simulink model "liner_control"  (R2019b)
settings: Solver=FixedStepAuto  StartTime=0.0  StopTime=100  FixedStep=0.01  RelTol=1e-3
undefined symbols (not defined in the file or in its folder): DiscIntNeverNeededParam
libraries: sbox2 x4, simulink x2
settings Model: Creator=haketa  LastModifiedBy=admin
settings DataIOCC: SaveFormat=Array  SignalLoggingSaveFormat=ModelDataLogs  ReturnWorkspaceOutputs=off
settings OptimizationCC: BlockReduction=off  OptimizeBlockIOStorage=off  BufferReuse=off  GlobalBufferReuse=off  ExpressionFolding=off  ExpressionDepthLimit=2147483647  LocalBlockOutputs=off  InitFltsAndDblsToZero=on  LifeSpan=inf  OptimizeDataStoreBuffers=off  BusAssignmentInplaceUpdate=off
settings DebuggingCC: SaveWithParameterizedLinksMsg=none  UnderspecifiedInitializationDetection=Classic  MergeDetectMultiDrivingBlocksExec=none  SignalResolutionControl=TryResolveAllWithWarning  SolverPrmCheckMsg=warning  InheritedTsInSrcMsg=none  MultiTaskDSMMsg=warning  MultiTaskCondExecSysMsg=none  FcnCallInpInsideContextMsg=warning  StateNameClashWarn=warning  SFUnexpectedBacktrackingDiag=warning  SFNoUnconditionalDefaultTransitionDiag=warning  SFExecutionAtInitializationDiag=none  ArithmeticOperatorsInVariantConditions=warning
settings HardwareCC: ProdBitPerPointer=32  ProdBitPerSizeT=32  ProdBitPerPtrDiffT=32  ProdLargestAtomicFloat=None  ProdIntDivRoundTo=Undefined  ProdEndianess=Unspecified  ProdWordSize=32  ProdHWDeviceType=32-bit Generic
settings ModelReferenceCC: PropagateSignalLabelsOutOfModel=off
settings SFSimCC: SimUseLocalCustomCode=off  CustomCodeUndefinedFunction=UseInterfaceOnly
settings RTWCC: Description=MTT sBOXII Real-Time Target.  SystemTargetFile=sbox2.tlc  TemplateMakefile=sbox2.tmf  RTWUseLocalCustomCode=off  RTWCompilerOptimization=on
settings CodeAppCC: StateflowObjectComments=on
settings GRTTargetCC: TargetLangStandard=C89/C90 (ANSI)  GeneratePreprocessorConditionals=Disable all  MatFileLogging=off  UseToolchainInfoCompliant=off  RTWCAPISignals=on  RTWCAPIParams=on
settings ConfigComp: CovMetricSettings=dw  CovHtmlReporting=on  CovSaveCumulativeToWorkspaceVar=on  CovSaveSingleToWorkspaceVar=on  CovExternalEMLEnable=off  CovSFcnEnable=off

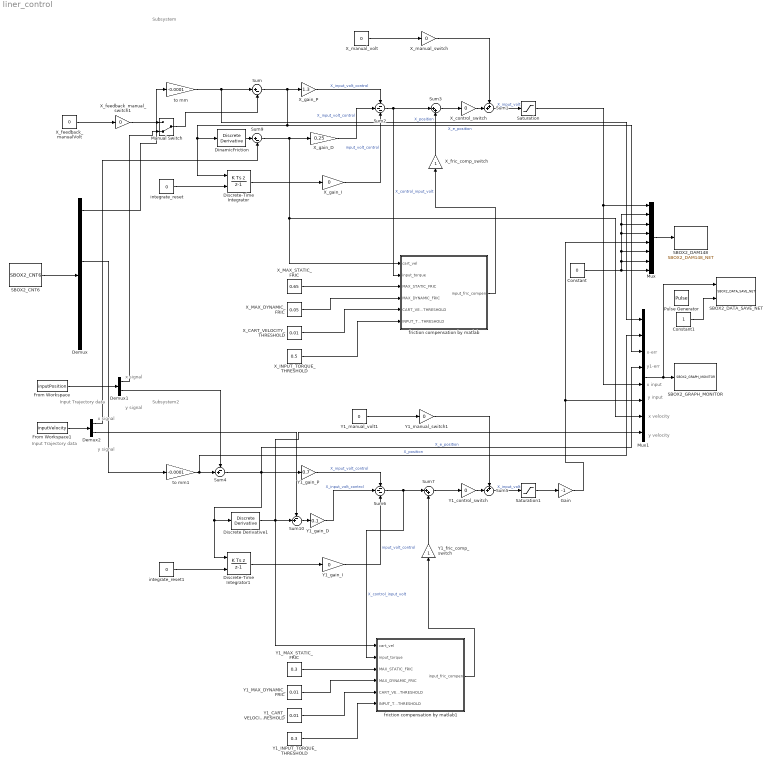
== system liner_control ==
  note: y velocity
  note: x velocity
  note: y input
  note: x input
  note: Input Trajectory data
  note: x signal
  note: y1-err
  note: x-err
  note: Subsystem2
  note: Subsystem
  note: y signal
  note: Input Trajectory data
  note: x signal
  note: y signal
  Constant : Constant  Value=0
  Constant1 : Constant
  Demux : Demux  Outputs=6
  Demux1 : Demux  Outputs=2
  Demux2 : Demux  Outputs=2
  DinamicFriction : simulink/Discrete/Discrete Derivative  gainval=1.0  ICPrevScaledInput=0.0  OutMin=[]  OutMax=[]  OutDataType=fixdt(1, 16)  OutScaling=2^-10  DoSatur=off
  Discrete Derivative1 : simulink/Discrete/Discrete Derivative  gainval=1.0  ICPrevScaledInput=0.0  OutMin=[]  OutMax=[]  OutDataType=fixdt(1, 16)  OutScaling=2^-10  DoSatur=off
  Discrete-Time Integrator : DiscreteIntegrator  IntegratorMethod=Integration: Backward Euler  ExternalReset=rising  SampleTime=-1  ICPrevOutput=DiscIntNeverNeededParam  ICPrevScaledInput=DiscIntNeverNeededParam
  Discrete-Time Integrator1 : DiscreteIntegrator  IntegratorMethod=Integration: Backward Euler  ExternalReset=rising  SampleTime=-1  ICPrevOutput=DiscIntNeverNeededParam  ICPrevScaledInput=DiscIntNeverNeededParam
  From Workspace : FromWorkspace  VariableName=inputPosition  SampleTime=0.01
  From Workspace1 : FromWorkspace  VariableName=inputVelocity  SampleTime=0.01
  Gain : Gain  Gain=-1
  Manual Switch : ManualSwitch  CurrentSetting=0
  Mux : Mux  Inputs=8
  Mux1 : Mux  Inputs=8
  Pulse Generator : DiscretePulseGenerator  Period=100  PulseWidth=5
  SBOX2_CNT6 : sbox2/Digital I//O Devices/SBOX2_CNT6  mode=2相パルス  teibai=x4  filter=off  zphase=動作なし  polarity=正論理 (high active)  mode2=2相パルス  teibai2=x4  filter2=off  zphase2=動作なし  polarity2=正論理 (high active)  mode3=2相パルス  teibai3=x4  filter3=off  zphase3=動作なし  polarity3=正論理 (high active)  mode4=2相パルス  teibai4=x4  filter4=off  zphase4=動作なし  polarity4=正論理 (high active)  mode5=2相パルス  teibai5=x4  filter5=off  zphase5=動作なし  polarity5=正論理 (high active)  mode6=2相パルス  teibai6=x4  filter6=off  zphase6=動作なし  polarity6=正論理 (high active)  dtype=FLOATING POINT  sampletime=-1
  "SBOX2_DAM148 " : sbox2/Analog I//O Devices/SBOX2_DAM148_NET  daStopCtrl1=DA出力継続  daStopCtrl2=DA出力継続  daStopCtrl3=DA出力継続  daStopCtrl4=DA出力継続  daStopCtrl5=DA出力継続  daStopCtrl6=DA出力継続  daStopCtrl7=DA出力継続  daStopCtrl8=DA出力継続  sampletime=-1
  SBOX2_DATA_SAVE_NET : sbox2/Network Data Save Devices/SBOX2_DATA_SAVE_NET  save_mode=ホストアプリケーション指示によるトリガ待ち  data_length=500  pre_triger=0  sampletime=-1
  SBOX2_GRAPH_MONITOR : sbox2/Network Data Save Devices/SBOX2_GRAPH_MONITOR  sampletime=-1
  Saturation : Saturate  UpperLimit=5  LowerLimit=-5
  Saturation1 : Saturate  UpperLimit=5  LowerLimit=-5
  Sum : Sum  Inputs=|+-
  Sum1 : Sum  Inputs=++|
  Sum10 : Sum  Inputs=-+|
  Sum2 : Sum  Inputs=---
  Sum3 : Sum  Inputs=|++
  Sum4 : Sum  Inputs=-+|
  Sum5 : Sum  Inputs=++|
  Sum6 : Sum  Inputs=---
  Sum7 : Sum  Inputs=|++
  Sum9 : Sum  Inputs=|+-
  X_CART_VELOCITY_THRESHOLD : Constant  Value=0.01
  X_INPUT_TORQUE_THRESHOLD : Constant  Value=0.5
  X_MAX_DYNAMIC_FRIC : Constant  Value=0.05
  X_MAX_STATIC_FRIC : Constant  Value=0.65
  X_control_switch : Gain  Gain=0
  X_feedback_manualVolt : Constant  Value=0
  X_feedback_manual_switch1 : Gain  Gain=0
  X_fric_comp_switch : Gain
  X_gain_D : Gain  Gain=0.25
  X_gain_I : Gain  Gain=0
  X_gain_P : Gain  Gain=1.3
  X_manual_switch : Gain  Gain=0
  X_manual_volt : Constant  Value=0
  Y1_CART_VELOCITY_THRESHOLD : Constant  Value=0.01
  Y1_INPUT_TORQUE_THRESHOLD : Constant  Value=0.3
  Y1_MAX_DYNAMIC_FRIC : Constant  Value=0.01
  Y1_MAX_STATIC_FRIC : Constant  Value=0.3
  Y1_control_switch : Gain  Gain=0
  Y1_fric_comp_switch : Gain
  Y1_gain_D : Gain  Gain=0.1
  Y1_gain_I : Gain  Gain=0
  Y1_gain_P : Gain  Gain=0.7
  Y1_manual_switch1 : Gain  Gain=0
  Y1_manual_volt1 : Constant  Value=0
  friction compensation by matlab : MATLAB Function  TreatAsAtomicUnit=on
  friction compensation by matlab1 : MATLAB Function  TreatAsAtomicUnit=on
  integrate_reset : Constant  Value=0
  integrate_reset1 : Constant  Value=0
  to mm : Gain  Gain=-0.0001
  to mm1 : Gain  Gain=-0.0001
  wires:
  SBOX2_CNT6/1 -> Demux/1
  Mux/1 -> "SBOX2_DAM148 "/1
  Constant/1 -> Mux/7, Mux/3, Mux/2, Mux/4, Mux/6, Mux/8
  Saturation/1 -> Mux1/5, Mux/1
  Saturation1/1 -> Gain/1
  X_fric_comp_switch/1 -> Sum3/2
  Sum3/1 -> X_control_switch/1
  X_manual_volt/1 -> X_manual_switch/1
  integrate_reset/1 -> Discrete-Time Integrator/2
  X_CART_VELOCITY_THRESHOLD/1 -> friction compensation by matlab/5(CART_VELOCITY_THRESHOLD)
  X_MAX_DYNAMIC_FRIC/1 -> friction compensation by matlab/4(MAX_DYNAMIC_FRIC)
  to mm/1 -> Mux1/1, Sum/1  "X_position"
  X_gain_D/1 -> Sum2/2  "X_input_volt_control"
  X_MAX_STATIC_FRIC/1 -> friction compensation by matlab/3(MAX_STATIC_FRIC)
  friction compensation by matlab/1(input_fric_compen) -> X_fric_comp_switch/1
  X_manual_switch/1 -> Sum1/1
  X_INPUT_TORQUE_THRESHOLD/1 -> friction compensation by matlab/6(INPUT_TORQUE_THRESHOLD)
  X_gain_I/1 -> Sum2/3  "input_volt_control"
  Sum/1 -> Mux1/3, DinamicFriction/1, Discrete-Time Integrator/1, X_gain_P/1  "X_e_position"
  X_gain_P/1 -> Sum2/1  "X_input_volt_control"
  Discrete-Time Integrator/1 -> X_gain_I/1
  Sum2/1 -> Sum3/1, friction compensation by matlab/2(input_torque)  "X_control_input_volt"
  Demux/1 -> to mm/1
  Sum9/1 -> friction compensation by matlab/1(cart_vel), Mux1/7, X_gain_D/1
  Sum1/1 -> Saturation/1  "X_input_volt"
  Y1_fric_comp_switch/1 -> Sum7/2
  Sum7/1 -> Y1_control_switch/1
  Y1_manual_volt1/1 -> Y1_manual_switch1/1
  integrate_reset1/1 -> Discrete-Time Integrator1/2
  Y1_CART_VELOCITY_THRESHOLD/1 -> friction compensation by matlab1/5(CART_VELOCITY_THRESHOLD)
  Y1_MAX_DYNAMIC_FRIC/1 -> friction compensation by matlab1/4(MAX_DYNAMIC_FRIC)
  to mm1/1 -> Sum4/2, Mux1/2  "X_position"
  Y1_gain_D/1 -> Sum6/2  "X_input_volt_control"
  Y1_MAX_STATIC_FRIC/1 -> friction compensation by matlab1/3(MAX_STATIC_FRIC)
  friction compensation by matlab1/1(input_fric_compen) -> Y1_fric_comp_switch/1
  Y1_manual_switch1/1 -> Sum5/1
  Y1_INPUT_TORQUE_THRESHOLD/1 -> friction compensation by matlab1/6(INPUT_TORQUE_THRESHOLD)
  Y1_gain_I/1 -> Sum6/3  "input_volt_control"
  Sum4/1 -> Discrete-Time Integrator1/1, Discrete Derivative1/1, Mux1/4, Y1_gain_P/1  "X_e_position"
  Y1_gain_P/1 -> Sum6/1  "X_input_volt_control"
  Discrete-Time Integrator1/1 -> Y1_gain_I/1
  Sum6/1 -> Sum7/1, friction compensation by matlab1/2(input_torque)  "X_control_input_volt"
  Demux/3 -> to mm1/1
  Discrete Derivative1/1 -> Sum10/2, friction compensation by matlab1/1(cart_vel), Mux1/8
  Sum5/1 -> Saturation1/1  "X_input_volt"
  Y1_control_switch/1 -> Sum5/2
  X_control_switch/1 -> Sum1/2
  Gain/1 -> Mux/5, Mux1/6
  From Workspace/1 -> Demux1/1
  Demux1/2 -> Sum4/1
  X_feedback_manual_switch1/1 -> Manual Switch/1
  X_feedback_manualVolt/1 -> X_feedback_manual_switch1/1
  Manual Switch/1 -> Sum/2
  Demux1/1 -> Manual Switch/2
  Mux1/1 -> SBOX2_GRAPH_MONITOR/1, SBOX2_DATA_SAVE_NET/1
  Constant1/1 -> SBOX2_DATA_SAVE_NET/2
  DinamicFriction/1 -> Sum9/1
  Demux2/1 -> Sum9/2
  From Workspace1/1 -> Demux2/1
  Demux2/2 -> Sum10/1
  Sum10/1 -> Y1_gain_D/1

== matlab function liner_control/friction compensation by matlab ==
  data: cart_vel input; input_fric_compen output; input_torque input; MAX_STATIC_FRIC input; MAX_DYNAMIC_FRIC input; CART_VELOCITY_THRESHOLD input; INPUT_TORQUE_THRESHOLD input
function input_fric_compen = fcn(cart_vel, input_torque, MAX_STATIC_FRIC, MAX_DYNAMIC_FRIC, CART_VELOCITY_THRESHOLD, INPUT_TORQUE_THRESHOLD)

input_fric_compen = zeros(1);

if abs(cart_vel) < CART_VELOCITY_THRESHOLD
    if input_torque > INPUT_TORQUE_THRESHOLD
        input_fric_compen = MAX_STATIC_FRIC * 0.9;
    else
        if input_torque < -INPUT_TORQUE_THRESHOLD
            input_fric_compen = - MAX_STATIC_FRIC * 0.9;
        else
            input_fric_compen = 0.0;
        end
    end
else
    if cart_vel > 0.0
        input_fric_compen = MAX_DYNAMIC_FRIC * 0.9;
    elseif cart_vel < 0.0
        input_fric_compen = - MAX_DYNAMIC_FRIC * 0.9;
    end
end

end

== matlab function liner_control/friction compensation by matlab1 ==
  data: cart_vel input; input_fric_compen output; input_torque input; MAX_STATIC_FRIC input; MAX_DYNAMIC_FRIC input; CART_VELOCITY_THRESHOLD input; INPUT_TORQUE_THRESHOLD input
function input_fric_compen = fcn(cart_vel, input_torque, MAX_STATIC_FRIC, MAX_DYNAMIC_FRIC, CART_VELOCITY_THRESHOLD, INPUT_TORQUE_THRESHOLD)

input_fric_compen = zeros(1);

if abs(cart_vel) < CART_VELOCITY_THRESHOLD
    if input_torque > INPUT_TORQUE_THRESHOLD
        input_fric_compen = MAX_STATIC_FRIC * 0.9;
    else
        if input_torque < -INPUT_TORQUE_THRESHOLD
            input_fric_compen = - MAX_STATIC_FRIC * 0.9;
        else
            input_fric_compen = 0.0;
        end
    end
else
    if cart_vel > 0.0
        input_fric_compen = MAX_DYNAMIC_FRIC * 0.9;
    elseif cart_vel < 0.0
        input_fric_compen = - MAX_DYNAMIC_FRIC * 0.9;
    end
end

end
